simulink model "demo"  (Simulink 7.5)
settings: Solver=ode5  StartTime=0.0  StopTime=60  FixedStep=0.001  RelTol=1e-3
libraries: mathlib x58, logiclib x37, execlib x12, reglib x12, genlib x8, anallib x4
settings Model: Creator=jsobota  LastModifiedBy=jsobota
settings SimMechanicsCC: VisOnUpdateDiagram=on

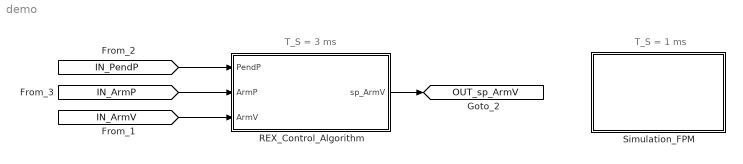
== system demo ==
  note: T_S = 3 ms
  note: T_S = 1 ms
  REX_Control_Algorithm : Subsystem  TreatAsAtomicUnit=on  SystemSampleTime=0.003
  Simulation_FPM : Subsystem  mask{g=9.81, r=0.3, l=0.23865, tau=0.06, rotate_sensor=-80*pi/180, alpha_pos0=0, alpha_vel0=0, beta_pos0=180*pi/180, beta_vel0=0}
      mask prompts: g "Gravity [m/s^2]"; r "Arm length [m]"; l "Pendulum length [m]"; tau "Velocity loop time constant"; rotate_sensor "Pendulum rotation sensor placement [rad]"; alpha_pos0 "Arm initial position [rad]"; alpha_vel0 "Arm initial velocity [rad/s]"; beta_pos0 "Pendulum initial position [rad]"; beta_vel0 "Pendulum initial velocity [rad/s]"
  tag scope: OUT_sp_ArmV=global
  wires:
  REX_Control_Algorithm/1(sp_ArmV) -> [OUT_sp_ArmV]
  [IN_PendP] -> REX_Control_Algorithm/1(PendP)
  [IN_ArmP] -> REX_Control_Algorithm/2(ArmP)
  [IN_ArmV] -> REX_Control_Algorithm/3(ArmV)

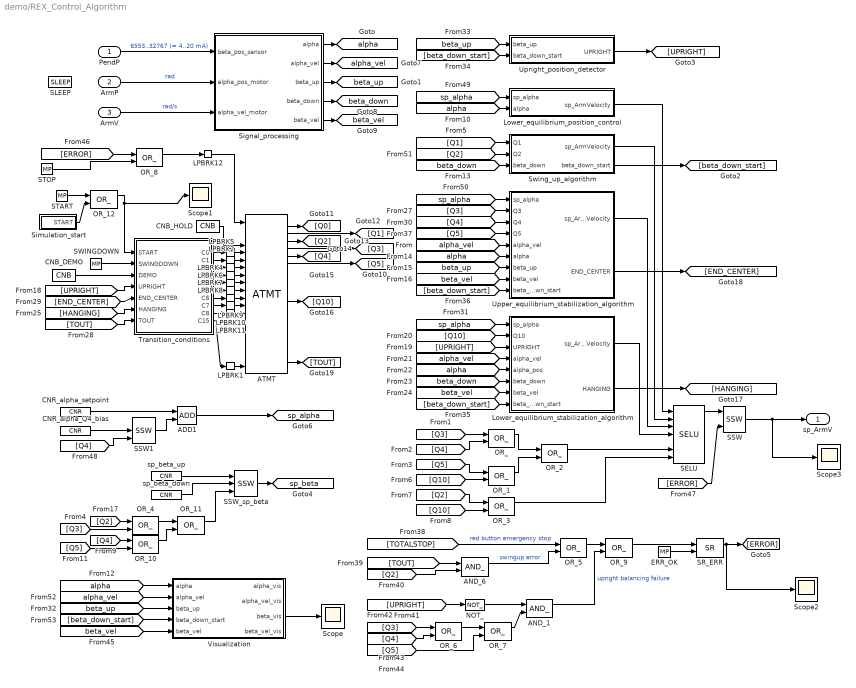
== system demo/REX_Control_Algorithm ==
  PendP : Inport
  ArmP : Inport  Port=2
  ArmV : Inport  Port=3
  ADD1 : mathlib/ADD  SystemSampleTime=-1
  AND_1 : logiclib/AND_  SystemSampleTime=-1
  AND_6 : logiclib/AND_  SystemSampleTime=-1
  ATMT : logiclib/ATMT  SystemSampleTime=-1  morestps=off  ntr=12  STT=[0 0 1;1 15 2;2 1 3;3 2 4;3 3 5;3 4 10;4 5 5;4 15 5;5 6 10;10 7 11;10 8 0;11 15 1]  touts=[0 0.5 1 20 10 10 0 0 0 0 5 5 0 0 0 0]
  CNB_DEMO : mathlib/CNB  SystemSampleTime=-1  YCN=on
  CNB_HOLD : mathlib/CNB  SystemSampleTime=-1  YCN=off
  CNR_alpha_Q4_bias : mathlib/CNR  SystemSampleTime=-1  ycn=3.1415
  CNR_alpha_setpoint : mathlib/CNR  SystemSampleTime=-1  ycn=0
  ERR_OK : genlib/MP  SystemSampleTime=-1  pwidth=0.01  BSTATE=off  RPTF=off
  LPBRK{1..2,4..12} (11 alike) : execlib/LPBRK
  Lower_equilibrium_position_control : Subsystem
      mask Type: REX sequence
  Lower_equilibrium_stabilization_algorithm : Subsystem
      mask Type: REX sequence
  NOT_ : logiclib/NOT_  SystemSampleTime=-1
  OR_{,1..12} (13 alike) : logiclib/OR_  SystemSampleTime=-1
  SELU : reglib/SELU  SystemSampleTime=-1  BINF=on
  SLEEP : execlib/SLEEP  SystemSampleTime=-1  ts=0
  SR_ERR : logiclib/SR  SystemSampleTime=-1
  SSW : reglib/SSW  SystemSampleTime=-1
  SSW1 : reglib/SSW  SystemSampleTime=-1
  SSW_sp_beta : reglib/SSW  SystemSampleTime=-1
  START : genlib/MP  SystemSampleTime=-1  pwidth=0.01  BSTATE=off  RPTF=off
  STOP : genlib/MP  SystemSampleTime=-1  pwidth=0.01  BSTATE=off  RPTF=off
  SWINGDOWN : genlib/MP  SystemSampleTime=-1  pwidth=0.01  BSTATE=off  RPTF=off
  Scope{,1..3} (4 alike) : Scope
      Scope settings: TimeRange=10  YMin=-4
      Scope1 settings: TimeRange=10  YMin=-4
      Scope2 settings: TimeRange=10  YMin=-4  SaveName=ScopeData2
      Scope3 settings: TimeRange=10  YMin=-4  SaveName=ScopeData3
  Signal_processing : Subsystem
      mask Type: REX sequence
  Simulation_start : Subsystem
  Swing_up_algorithm : Subsystem
      mask Type: REX sequence
  Transition_conditions : Subsystem
  Upper_equilibrium_stabilization_algorithm : Subsystem
      mask Type: REX sequence
  Upright_position_detector : Subsystem
  Visualization : Subsystem
  sp_beta_down : mathlib/CNR  SystemSampleTime=-1  ycn=3.1415
  sp_beta_up : mathlib/CNR  SystemSampleTime=-1  ycn=0
  sp_ArmV : Outport
  tag scope: alpha=global, alpha_vel=global, beta_down=global, beta_up=global, beta_vel=global, sp_alpha=global, sp_beta=global
  wires:
  ATMT/1 -> [Q0]
  ATMT/2 -> [Q1]
  ATMT/3 -> [Q2]
  ATMT/4 -> [Q3]
  ATMT/5 -> [Q4]
  ATMT/11 -> [Q10]
  ATMT/19 -> [TOUT]
  [alpha_vel] -> Upper_equilibrium_stabilization_algorithm/5(alpha_vel)
  [Q3] -> OR_/1
  [alpha] -> Lower_equilibrium_position_control/2(alpha)
  [beta_down] -> Swing_up_algorithm/3(beta_down)
  [alpha] -> Upper_equilibrium_stabilization_algorithm/6(alpha)
  [beta_up] -> Upper_equilibrium_stabilization_algorithm/7(beta_up)
  [beta_vel] -> Upper_equilibrium_stabilization_algorithm/8(beta_vel)
  [UPRIGHT] -> Lower_equilibrium_stabilization_algorithm/3(UPRIGHT)
  [Q4] -> OR_/2
  [Q10] -> Lower_equilibrium_stabilization_algorithm/2(Q10)
  [alpha_vel] -> Lower_equilibrium_stabilization_algorithm/4(alpha_vel)
  [alpha] -> Lower_equilibrium_stabilization_algorithm/5(alpha_pos)
  [beta_down] -> Lower_equilibrium_stabilization_algorithm/6(beta_down)
  [beta_vel] -> Lower_equilibrium_stabilization_algorithm/7(beta_vel)
  [Q3] -> Upper_equilibrium_stabilization_algorithm/2(Q3)
  [Q5] -> OR_1/1
  [Q10] -> OR_1/2
  [Q2] -> OR_3/1
  [Q10] -> OR_3/2
  ArmV/1 -> Signal_processing/3(alpha_vel_motor)  "rad/s"
  PendP/1 -> Signal_processing/1(beta_pos_sensor)  "6553..32767 (= 4..20 mA)"
  CNB_HOLD/1 -> ATMT/4
  LPBRK1/1 -> ATMT/20
  Lower_equilibrium_position_control/1(sp_ArmVelocity) -> SELU/1
  Lower_equilibrium_stabilization_algorithm/1(sp_ArmVelocity) -> SELU/4
  Lower_equilibrium_stabilization_algorithm/2(HANGING) -> [HANGING]
  OR_/1 -> OR_2/1
  OR_1/1 -> OR_2/2
  OR_2/1 -> SELU/6
  OR_3/1 -> SELU/7
  Signal_processing/1(alpha) -> [alpha]
  Signal_processing/2(alpha_vel) -> [alpha_vel]
  Signal_processing/3(beta_up) -> [beta_up]
  Signal_processing/4(beta_down) -> [beta_down]
  Signal_processing/5(beta_vel) -> [beta_vel]
  Swing_up_algorithm/1(sp_ArmVelocity) -> SELU/2
  Swing_up_algorithm/2(beta_down_start) -> [beta_down_start]
  Upper_equilibrium_stabilization_algorithm/1(sp_ArmVelocity) -> SELU/3
  ArmP/1 -> Signal_processing/2(alpha_pos_motor)  "rad"
  Upper_equilibrium_stabilization_algorithm/2(END_CENTER) -> [END_CENTER]
  [Q4] -> Upper_equilibrium_stabilization_algorithm/3(Q4)
  Upright_position_detector/1(UPRIGHT) -> [UPRIGHT]
  [beta_up] -> Upright_position_detector/1(beta_up)
  [beta_down_start] -> Upright_position_detector/2(beta_down_start)
  [beta_down_start] -> Lower_equilibrium_stabilization_algorithm/8(beta_down_start)
  [beta_down_start] -> Upper_equilibrium_stabilization_algorithm/9(beta_down_start)
  [Q5] -> Upper_equilibrium_stabilization_algorithm/4(Q5)
  [TOUT] -> AND_6/1
  [Q2] -> AND_6/2
  [UPRIGHT] -> NOT_/1
  [Q3] -> OR_6/1
  [Q4] -> OR_6/2
  [Q5] -> OR_7/2
  OR_6/1 -> OR_7/1
  OR_7/1 -> AND_1/2
  NOT_/1 -> AND_1/1
  AND_1/1 -> OR_9/2  "upright balancing failure"
  [TOTALSTOP] -> OR_5/1  "red button emergency stop"
  AND_6/1 -> OR_5/2  "swingup error"
  ERR_OK/1 -> SR_ERR/2
  SR_ERR/1 -> [ERROR], Scope2/1
  [ERROR] -> OR_8/1
  STOP/1 -> OR_8/2
  OR_8/1 -> LPBRK12/1
  SELU/1 -> SSW/1
  SSW/1 -> sp_ArmV/1, Scope3/1
  [ERROR] -> SSW/3
  CNR_alpha_setpoint/1 -> ADD1/1
  SSW1/1 -> ADD1/2
  [Q4] -> SSW1/3
  CNR_alpha_Q4_bias/1 -> SSW1/2
  ADD1/1 -> [sp_alpha]
  [sp_alpha] -> Lower_equilibrium_position_control/1(sp_alpha)
  [sp_alpha] -> Upper_equilibrium_stabilization_algorithm/1(sp_alpha)
  [Q1] -> Swing_up_algorithm/1(Q1)
  [Q2] -> Swing_up_algorithm/2(Q2)
  ATMT/6 -> [Q5]
  OR_5/1 -> OR_9/1
  OR_9/1 -> SR_ERR/1
  Transition_conditions/10(C15) -> LPBRK1/1
  CNB_DEMO/1 -> Transition_conditions/3(DEMO)
  SWINGDOWN/1 -> Transition_conditions/2(SWINGDOWN)
  START/1 -> OR_12/1
  [UPRIGHT] -> Transition_conditions/4(UPRIGHT)
  [END_CENTER] -> Transition_conditions/5(END_CENTER)
  [HANGING] -> Transition_conditions/6(HANGING)
  [TOUT] -> Transition_conditions/7(TOUT)
  Transition_conditions/1(C0) -> LPBRK5/1
  LPBRK5/1 -> ATMT/5
  Transition_conditions/2(C1) -> LPBRK2/1
  Transition_conditions/3(C2) -> LPBRK4/1
  Transition_conditions/4(C3) -> LPBRK6/1
  Transition_conditions/5(C4) -> LPBRK7/1
  Transition_conditions/6(C5) -> LPBRK8/1
  Transition_conditions/7(C6) -> LPBRK9/1
  Transition_conditions/8(C7) -> LPBRK10/1
  Transition_conditions/9(C8) -> LPBRK11/1
  LPBRK12/1 -> ATMT/1
  [sp_alpha] -> Lower_equilibrium_stabilization_algorithm/1(sp_alpha)
  Simulation_start/1(START) -> OR_12/2
  LPBRK2/1 -> ATMT/6
  LPBRK4/1 -> ATMT/7
  LPBRK6/1 -> ATMT/8
  LPBRK7/1 -> ATMT/9
  LPBRK8/1 -> ATMT/10
  LPBRK9/1 -> ATMT/11
  LPBRK10/1 -> ATMT/12
  LPBRK11/1 -> ATMT/13
  [alpha] -> Visualization/1(alpha)
  [alpha_vel] -> Visualization/2(alpha_vel)
  [beta_up] -> Visualization/3(beta_up)
  [beta_down_start] -> Visualization/4(beta_down_start)
  [beta_vel] -> Visualization/5(beta_vel)
  Visualization/3(beta_vis) -> Scope/1
  sp_beta_up/1 -> SSW_sp_beta/1
  sp_beta_down/1 -> SSW_sp_beta/2
  [Q2] -> OR_4/1
  [Q3] -> OR_4/2
  [Q4] -> OR_10/1
  [Q5] -> OR_10/2
  OR_4/1 -> OR_11/1
  OR_10/1 -> OR_11/2
  OR_11/1 -> SSW_sp_beta/3
  SSW_sp_beta/1 -> [sp_beta]
  OR_12/1 -> Transition_conditions/1(START), Scope1/1

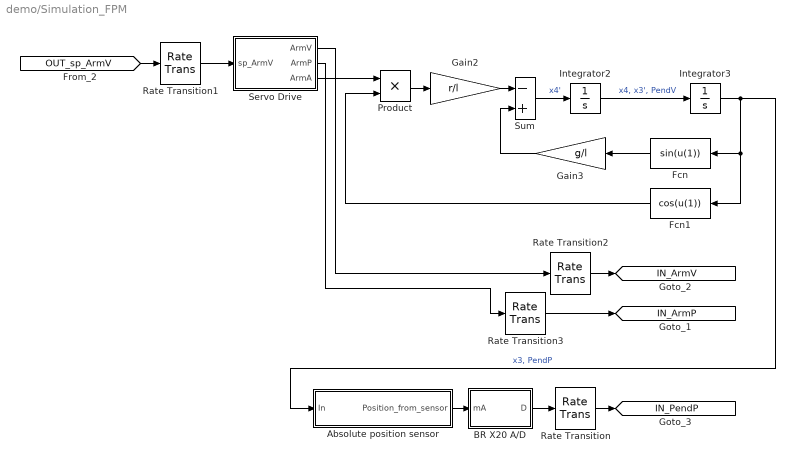
== system demo/Simulation_FPM ==
  Absolute position sensor : Subsystem
  BR X20 A/D : Subsystem
  Fcn : Fcn  Expr=sin(u(1))
  Fcn1 : Fcn  Expr=cos(u(1))
  Gain2 : Gain  Gain=r/l  ParameterDataType=fixdt(1, 16)  ParameterScaling=2^0  OutDataType=fixdt(1, 16)  OutScaling=2^0
  Gain3 : Gain  Gain=g/l  ParameterDataType=fixdt(1, 16)  ParameterScaling=2^0  OutDataType=fixdt(1, 16)  OutScaling=2^0
  Integrator2 : Integrator  InitialCondition=beta_vel0
  Integrator3 : Integrator  InitialCondition=beta_pos0
  Product : Product  OutDataType=fixdt(1, 16)  OutScaling=2^0  RndMeth=Zero
  Rate Transition : RateTransition  Integrity=off  OutPortSampleTimeOpt=Inherit  OutPortSampleTime=0.1
  Rate Transition1 : RateTransition  Integrity=off  Deterministic=off  OutPortSampleTimeOpt=Inherit
  Rate Transition2 : RateTransition  Integrity=off  OutPortSampleTimeOpt=Inherit  OutPortSampleTime=0.1
  Rate Transition3 : RateTransition  Integrity=off  OutPortSampleTimeOpt=Inherit  OutPortSampleTime=0.1
  Servo Drive : Subsystem
  Sum : Sum  Inputs=-+  OutDataType=fixdt(1, 16)  OutScaling=2^0
  tag scope: IN_ArmP=global, IN_ArmV=global, IN_PendP=global
  wires:
  Sum/1 -> Integrator2/1  "x4'"
  Integrator2/1 -> Integrator3/1  "x4, x3', PendV"
  Integrator3/1 -> Absolute position sensor/1(In), Fcn/1, Fcn1/1  "x3, PendP"
  Gain3/1 -> Sum/2
  Fcn/1 -> Gain3/1
  Fcn1/1 -> Product/2
  Product/1 -> Gain2/1
  Gain2/1 -> Sum/1
  Servo Drive/2(ArmP) -> Rate Transition3/1
  [OUT_sp_ArmV] -> Rate Transition1/1
  Rate Transition1/1 -> Servo Drive/1(sp_ArmV)
  Rate Transition/1 -> [IN_PendP]
  Rate Transition2/1 -> [IN_ArmV]
  Rate Transition3/1 -> [IN_ArmP]
  Servo Drive/1(ArmV) -> Rate Transition2/1
  Servo Drive/3(ArmA) -> Product/1
  Absolute position sensor/1(Position_from_sensor) -> BR X20 A/D/1(mA)
  BR X20 A/D/1(D) -> Rate Transition/1

== system demo/REX_Control_Algorithm/Lower_equilibrium_position_control ==
  sp_alpha : Inport
  alpha : Inport  Port=2
  GAIN_P_controller : mathlib/GAIN  SystemSampleTime=-1  k=2
  SUB : mathlib/SUB  SystemSampleTime=-1
  sp_ArmVelocity : Outport
  wires:
  GAIN_P_controller/1 -> sp_ArmVelocity/1
  SUB/1 -> GAIN_P_controller/1
  alpha/1 -> SUB/2
  sp_alpha/1 -> SUB/1

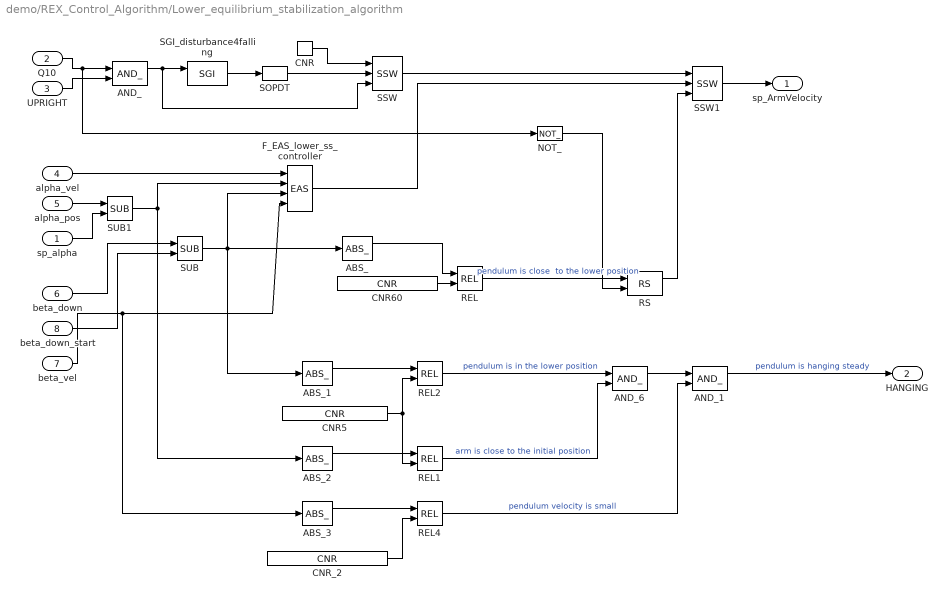
== system demo/REX_Control_Algorithm/Lower_equilibrium_stabilization_algorithm ==
  sp_alpha : Inport
  Q10 : Inport  Port=2
  UPRIGHT : Inport  Port=3
  alpha_vel : Inport  Port=4
  alpha_pos : Inport  Port=5
  beta_down : Inport  Port=6  OutDataType=sfix(16)  OutScaling=2^0
  beta_vel : Inport  Port=7  OutDataType=sfix(16)  OutScaling=2^0
  beta_down_start : Inport  Port=8  OutDataType=sfix(16)  OutScaling=2^0
  ABS_{,1..3} (4 alike) : mathlib/ABS_  SystemSampleTime=-1
  AND_ : logiclib/AND_  SystemSampleTime=-1
  AND_1 : logiclib/AND_  SystemSampleTime=-1
  AND_6 : logiclib/AND_  SystemSampleTime=-1
  CNR : mathlib/CNR  SystemSampleTime=-1  ycn=0
  CNR5 : mathlib/CNR  SystemSampleTime=-1  ycn=0.087266462599716
  CNR60 : mathlib/CNR  SystemSampleTime=-1  ycn=0.5
  CNR_2 : mathlib/CNR  SystemSampleTime=-1  ycn=0.0017453292519943
  F_EAS_lower_ss_controller : mathlib/EAS  SystemSampleTime=-1  a=6.12354219E-001  b=-4.25163230E-001  c=-2.53804417E+000  d=-3.30908089E-001  y0=0
  NOT_ : logiclib/NOT_  SystemSampleTime=-1
  REL{,1..2,4} (4 alike) : mathlib/REL  SystemSampleTime=-1  irel=3: less than (<)
  RS : logiclib/RS  SystemSampleTime=-1
  SGI_disturbance4falling : genlib/SGI  SystemSampleTime=-1  isig=4: RANDOM  amp=1  freq=1  phase=0  ifrunit=1: Hz  iphunit=1: degrees
  SOPDT : reglib/SOPDT  SystemSampleTime=-1  itf=2: Real poles  k0=1  tau=0  tau1=0.1  tau2=0.2  om=1  xi=1  pb0=1  pb1=1  pa0=1  pa1=1  del=0
  SSW : reglib/SSW  SystemSampleTime=-1
  SSW1 : reglib/SSW  SystemSampleTime=-1
  SUB : mathlib/SUB  SystemSampleTime=-1
  SUB1 : mathlib/SUB  SystemSampleTime=-1
  sp_ArmVelocity : Outport
  HANGING : Outport  Port=2
  wires:
  ABS_/1 -> REL/1
  ABS_1/1 -> REL2/1
  ABS_2/1 -> REL1/1
  ABS_3/1 -> REL4/1
  AND_/1 -> SGI_disturbance4falling/1, SSW/3
  AND_1/1 -> HANGING/1  "pendulum is hanging steady"
  AND_6/1 -> AND_1/1
  CNR/1 -> SSW/1
  CNR5/1 -> REL1/2, REL2/2
  CNR60/1 -> REL/2
  CNR_2/1 -> REL4/2
  F_EAS_lower_ss_controller/1 -> SSW1/2
  NOT_/1 -> RS/2
  Q10/1 -> AND_/1, NOT_/1
  REL/1 -> RS/1  "pendulum is close  to the lower position"
  REL1/1 -> AND_6/2  "arm is close to the initial position"
  REL2/1 -> AND_6/1  "pendulum is in the lower position"
  REL4/1 -> AND_1/2  "pendulum velocity is small"
  RS/1 -> SSW1/3
  SGI_disturbance4falling/1 -> SOPDT/1
  SOPDT/1 -> SSW/2
  SSW/1 -> SSW1/1
  SSW1/1 -> sp_ArmVelocity/1
  SUB/1 -> ABS_/1, ABS_1/1, F_EAS_lower_ss_controller/3
  UPRIGHT/1 -> AND_/2
  alpha_pos/1 -> SUB1/1
  alpha_vel/1 -> F_EAS_lower_ss_controller/1
  beta_down/1 -> SUB/1
  beta_down_start/1 -> SUB/2
  beta_vel/1 -> ABS_3/1, F_EAS_lower_ss_controller/4
  SUB1/1 -> ABS_2/1, F_EAS_lower_ss_controller/2
  sp_alpha/1 -> SUB1/2

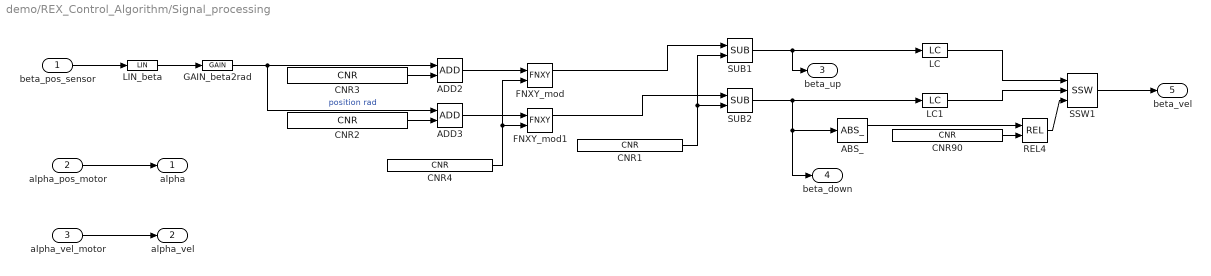
== system demo/REX_Control_Algorithm/Signal_processing ==
  beta_pos_sensor : Inport
  alpha_pos_motor : Inport  Port=2
  alpha_vel_motor : Inport  Port=3
  ABS_ : mathlib/ABS_  SystemSampleTime=-1
  ADD2 : mathlib/ADD  SystemSampleTime=-1
  ADD3 : mathlib/ADD  SystemSampleTime=-1
  CNR1 : mathlib/CNR  SystemSampleTime=-1  ycn=3.14159265358979
  CNR2 : mathlib/CNR  SystemSampleTime=-1  ycn=4.71238898038469
  CNR3 : mathlib/CNR  SystemSampleTime=-1  ycn=7.853981633974483
  CNR4 : mathlib/CNR  SystemSampleTime=-1  ycn=6.283185307179586
  CNR90 : mathlib/CNR  SystemSampleTime=-1  ycn=1.570796326794897
  FNXY_mod : mathlib/FNXY  SystemSampleTime=-1  ifn=2: fmod  yerr=0.0
  FNXY_mod1 : mathlib/FNXY  SystemSampleTime=-1  ifn=2: fmod  yerr=0.0
  GAIN_beta2rad : mathlib/GAIN  SystemSampleTime=-1  k=0.0175
  LC : reglib/LC  SystemSampleTime=-1  td=1  nd=30  ISSF=off
  LC1 : reglib/LC  SystemSampleTime=-1  td=1  nd=30  ISSF=off
  LIN_beta : mathlib/LIN  SystemSampleTime=-1  u1=6553  y1=5  u2=32767  y2=355
  REL4 : mathlib/REL  SystemSampleTime=-1  irel=3: less than (<)
  SSW1 : reglib/SSW  SystemSampleTime=-1
  SUB1 : mathlib/SUB  SystemSampleTime=-1
  SUB2 : mathlib/SUB  SystemSampleTime=-1
  alpha : Outport
  alpha_vel : Outport  Port=2
  beta_up : Outport  Port=3
  beta_down : Outport  Port=4
  beta_vel : Outport  Port=5
  wires:
  ABS_/1 -> REL4/1
  ADD2/1 -> FNXY_mod/1
  ADD3/1 -> FNXY_mod1/1
  CNR1/1 -> SUB1/2, SUB2/2
  CNR2/1 -> ADD3/2
  CNR3/1 -> ADD2/2
  CNR4/1 -> FNXY_mod/2, FNXY_mod1/2
  CNR90/1 -> REL4/2
  FNXY_mod/1 -> SUB1/1
  FNXY_mod1/1 -> SUB2/1
  GAIN_beta2rad/1 -> ADD2/1, ADD3/1  "position rad"
  LC/1 -> SSW1/1
  LC1/1 -> SSW1/2
  REL4/1 -> SSW1/3
  SSW1/1 -> beta_vel/1
  SUB1/1 -> LC/1, beta_up/1
  SUB2/1 -> ABS_/1, beta_down/1, LC1/1
  alpha_vel_motor/1 -> alpha_vel/1
  LIN_beta/1 -> GAIN_beta2rad/1
  beta_pos_sensor/1 -> LIN_beta/1
  alpha_pos_motor/1 -> alpha/1

== system demo/REX_Control_Algorithm/Simulation_start ==
  BIS : genlib/BIS  SystemSampleTime=-1  Y0=off  t1=5  t2=6  t3=0  t4=4  t5=5  t6=6  t7=7  t8=8  RPT=off
  START : Outport
  wires:
  BIS/1 -> START/1

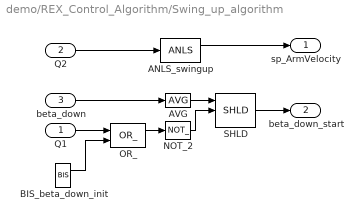
== system demo/REX_Control_Algorithm/Swing_up_algorithm ==
  Q1 : Inport
  Q2 : Inport  Port=2
  beta_down : Inport  Port=3  OutDataType=sfix(16)  OutScaling=2^0
  ANLS_swingup : genlib/ANLS  SystemSampleTime=-1  y0=-10  t1=0.226  y1=-10  t2=0.226  y2=10  t3=1  y3=10  t4=1  y4=0  RPT=off
  AVG : anallib/AVG  SystemSampleTime=-1  n=100
  BIS_beta_down_init : genlib/BIS  SystemSampleTime=-1  Y0=off  t1=1  t2=2  t3=0  t4=4  t5=5  t6=6  t7=7  t8=8  RPT=off
  NOT_2 : logiclib/NOT_  SystemSampleTime=-1
  OR_ : logiclib/OR_  SystemSampleTime=-1
  SHLD : anallib/SHLD  SystemSampleTime=-1  y0=0
  sp_ArmVelocity : Outport
  beta_down_start : Outport  Port=2
  wires:
  ANLS_swingup/1 -> sp_ArmVelocity/1
  AVG/1 -> SHLD/1
  NOT_2/1 -> SHLD/2
  Q2/1 -> ANLS_swingup/1
  SHLD/1 -> beta_down_start/1
  beta_down/1 -> AVG/1
  Q1/1 -> OR_/1
  BIS_beta_down_init/1 -> OR_/2
  OR_/1 -> NOT_2/1

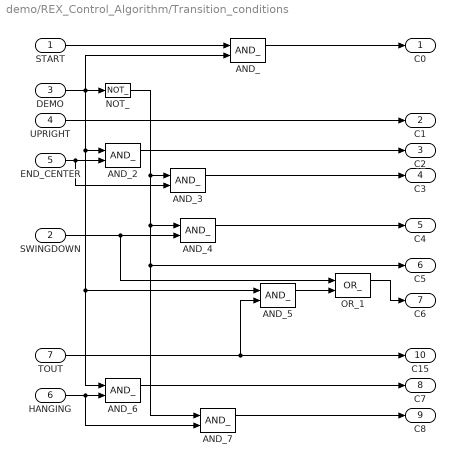
== system demo/REX_Control_Algorithm/Transition_conditions ==
  START : Inport
  SWINGDOWN : Inport  Port=2
  DEMO : Inport  Port=3
  UPRIGHT : Inport  Port=4
  END_CENTER : Inport  Port=5
  HANGING : Inport  Port=6
  TOUT : Inport  Port=7
  AND_{,2..7} (7 alike) : logiclib/AND_  SystemSampleTime=-1
  NOT_ : logiclib/NOT_  SystemSampleTime=-1
  OR_1 : logiclib/OR_  SystemSampleTime=-1
  C0 : Outport
  C1 : Outport  Port=2
  C2 : Outport  Port=3
  C3 : Outport  Port=4
  C4 : Outport  Port=5
  C5 : Outport  Port=6
  C6 : Outport  Port=7
  C7 : Outport  Port=8
  C8 : Outport  Port=9
  C15 : Outport  Port=10
  wires:
  START/1 -> AND_/1
  DEMO/1 -> AND_/2, NOT_/1, AND_2/1, AND_5/1, AND_6/1
  AND_/1 -> C0/1
  NOT_/1 -> AND_3/1, AND_4/1, C5/1, AND_7/1
  TOUT/1 -> C15/1, AND_5/2
  UPRIGHT/1 -> C1/1
  END_CENTER/1 -> AND_2/2, AND_3/2
  AND_2/1 -> C2/1
  AND_3/1 -> C3/1
  SWINGDOWN/1 -> AND_4/2, OR_1/1
  AND_4/1 -> C4/1
  AND_5/1 -> OR_1/2
  OR_1/1 -> C6/1
  HANGING/1 -> AND_6/2, AND_7/2
  AND_6/1 -> C7/1
  AND_7/1 -> C8/1

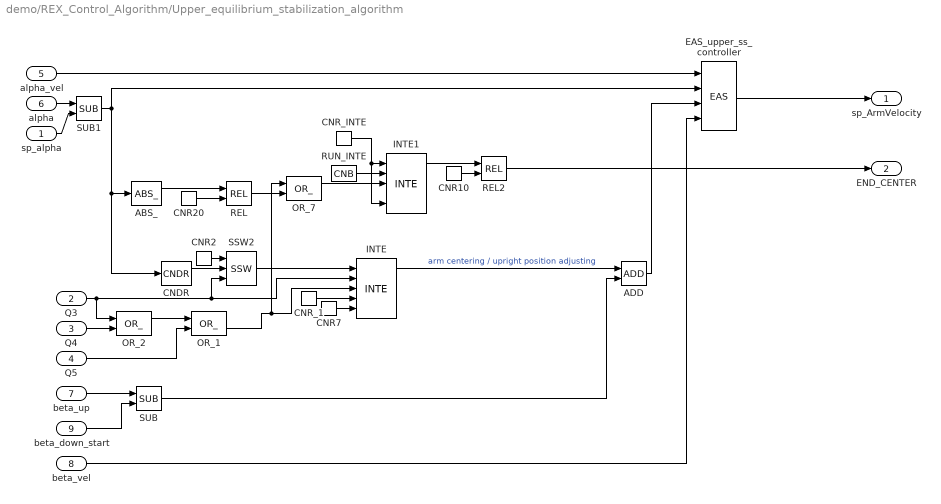
== system demo/REX_Control_Algorithm/Upper_equilibrium_stabilization_algorithm ==
  sp_alpha : Inport
  Q3 : Inport  Port=2
  Q4 : Inport  Port=3
  Q5 : Inport  Port=4
  alpha_vel : Inport  Port=5
  alpha : Inport  Port=6
  beta_up : Inport  Port=7  OutDataType=sfix(16)  OutScaling=2^0
  beta_vel : Inport  Port=8  OutDataType=sfix(16)  OutScaling=2^0
  beta_down_start : Inport  Port=9  OutDataType=sfix(16)  OutScaling=2^0
  ABS_ : mathlib/ABS_  SystemSampleTime=-1
  ADD : mathlib/ADD  SystemSampleTime=-1
  CNDR : reglib/CNDR  SystemSampleTime=-1  n=6  SATF=on  up=[-1.5708 -0.7854 -0.0523 0.0523 0.7854 1.5708]  yp=[-0.12 -0.04 0 0 0.04 0.12]
  CNR10 : mathlib/CNR  SystemSampleTime=-1  ycn=20
  CNR2 : mathlib/CNR  SystemSampleTime=-1  ycn=0
  CNR20 : mathlib/CNR  SystemSampleTime=-1  ycn=0.349065850398866
  CNR7 : mathlib/CNR  SystemSampleTime=-1  ycn=20
  CNR_1 : mathlib/CNR  SystemSampleTime=-1  ycn=0
  CNR_INTE : mathlib/CNR  SystemSampleTime=-1  ycn=1
  EAS_upper_ss_controller : mathlib/EAS  SystemSampleTime=-1  a=1.173059924  b=.1334856247  c=4.815526508  d=.7295211418  y0=0
  INTE : anallib/INTE  SystemSampleTime=-1  ymin=-1  ymax=1
  INTE1 : anallib/INTE  SystemSampleTime=-1  ymin=0  ymax=30
  OR_1 : logiclib/OR_  SystemSampleTime=-1
  OR_2 : logiclib/OR_  SystemSampleTime=-1
  OR_7 : logiclib/OR_  SystemSampleTime=-1
  REL : mathlib/REL  SystemSampleTime=-1  irel=4: greater than (>)
  REL2 : mathlib/REL  SystemSampleTime=-1  irel=4: greater than (>)
  RUN_INTE : mathlib/CNB  SystemSampleTime=-1  YCN=on
  SSW2 : reglib/SSW  SystemSampleTime=-1
  SUB : mathlib/SUB  SystemSampleTime=-1
  SUB1 : mathlib/SUB  SystemSampleTime=-1
  sp_ArmVelocity : Outport
  END_CENTER : Outport  Port=2
  wires:
  ABS_/1 -> REL/1
  ADD/1 -> EAS_upper_ss_controller/3
  CNDR/1 -> SSW2/2
  CNR10/1 -> REL2/2
  CNR2/1 -> SSW2/1
  CNR20/1 -> REL/2
  CNR7/1 -> INTE/5
  CNR_1/1 -> INTE/4
  CNR_INTE/1 -> INTE1/1, INTE1/5
  EAS_upper_ss_controller/1 -> sp_ArmVelocity/1
  INTE/1 -> ADD/1  "arm centering / upright position adjusting"
  INTE1/1 -> REL2/1
  OR_1/2 -> INTE/3, OR_7/1
  OR_7/1 -> INTE1/3
  Q3/1 -> SSW2/3, INTE/2, OR_2/1
  REL/1 -> OR_7/2
  RUN_INTE/1 -> INTE1/2
  SSW2/1 -> INTE/1
  SUB/1 -> ADD/2
  SUB1/1 -> ABS_/1, CNDR/1, EAS_upper_ss_controller/2
  alpha_vel/1 -> EAS_upper_ss_controller/1
  beta_down_start/1 -> SUB/2
  beta_up/1 -> SUB/1
  beta_vel/1 -> EAS_upper_ss_controller/4
  REL2/1 -> END_CENTER/1
  Q4/1 -> OR_2/2
  Q5/1 -> OR_1/2
  OR_2/1 -> OR_1/1
  alpha/1 -> SUB1/1
  sp_alpha/1 -> SUB1/2

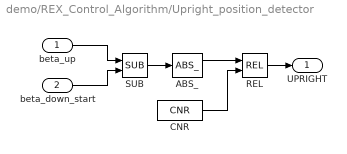
== system demo/REX_Control_Algorithm/Upright_position_detector ==
  beta_up : Inport
  beta_down_start : Inport  Port=2
  ABS_ : mathlib/ABS_  SystemSampleTime=-1
  CNR : mathlib/CNR  SystemSampleTime=-1  ycn=0.9
  REL : mathlib/REL  SystemSampleTime=-1  irel=3: less than (<)
  SUB : mathlib/SUB  SystemSampleTime=-1
  UPRIGHT : Outport
  wires:
  ABS_/1 -> REL/1
  CNR/1 -> REL/2
  SUB/1 -> ABS_/1
  beta_up/1 -> SUB/1
  REL/1 -> UPRIGHT/1
  beta_down_start/1 -> SUB/2

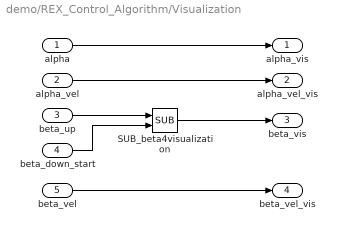
== system demo/REX_Control_Algorithm/Visualization ==
  alpha : Inport
  alpha_vel : Inport  Port=2
  beta_up : Inport  Port=3
  beta_down_start : Inport  Port=4
  beta_vel : Inport  Port=5
  SUB_beta4visualization : mathlib/SUB  SystemSampleTime=-1
  alpha_vis : Outport
  alpha_vel_vis : Outport  Port=2
  beta_vis : Outport  Port=3
  beta_vel_vis : Outport  Port=4
  wires:
  beta_up/1 -> SUB_beta4visualization/1
  beta_down_start/1 -> SUB_beta4visualization/2
  alpha/1 -> alpha_vis/1
  SUB_beta4visualization/1 -> beta_vis/1
  beta_vel/1 -> beta_vel_vis/1
  alpha_vel/1 -> alpha_vel_vis/1

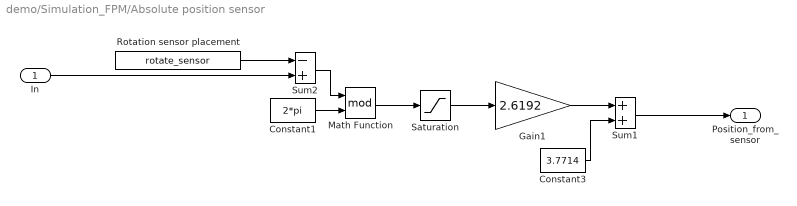
== system demo/Simulation_FPM/Absolute position sensor ==
  In : Inport
  Constant1 : Constant  Value=2*pi  OutDataType=fixdt(1, 16)  OutScaling=2^0
  Constant3 : Constant  Value=3.7714  OutDataType=fixdt(1, 16)  OutScaling=2^0
  Gain1 : Gain  Gain=2.6192  ParameterDataType=fixdt(1, 16)  ParameterScaling=2^0  OutDataType=fixdt(1, 16)  OutScaling=2^0
  Math Function : Math  Operator=mod  OutDataType=fixdt(1, 16)  OutScaling=2^0  SaturateOnIntegerOverflow=on
  Rotation sensor placement : Constant  Value=rotate_sensor  OutDataType=fixdt(1, 16)  OutScaling=2^0
  Saturation : Saturate  UpperLimit=355*pi/180  LowerLimit=5*pi/180  OutDataType=fixdt(1, 16)  OutScaling=2^0
  Sum1 : Sum  OutDataType=fixdt(1, 16)  OutScaling=2^0
  Sum2 : Sum  Inputs=-+  OutDataType=fixdt(1, 16)  OutScaling=2^0
  Position_from_sensor : Outport
  wires:
  Sum2/1 -> Math Function/1
  Rotation sensor placement/1 -> Sum2/1
  Math Function/1 -> Saturation/1
  Saturation/1 -> Gain1/1
  Constant1/1 -> Math Function/2
  In/1 -> Sum2/2
  Gain1/1 -> Sum1/1
  Constant3/1 -> Sum1/2
  Sum1/1 -> Position_from_sensor/1

== system demo/Simulation_FPM/BR X20 A/D ==
  mA : Inport
  Gain : Gain  Gain=1638.25  ParameterDataType=fixdt(1, 16)  ParameterScaling=2^0  OutDataType=fixdt(1, 16)  OutScaling=2^0
  D : Outport
  wires:
  mA/1 -> Gain/1
  Gain/1 -> D/1

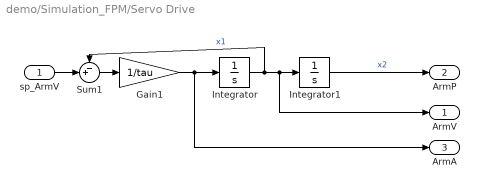
== system demo/Simulation_FPM/Servo Drive ==
  sp_ArmV : Inport
  Gain1 : Gain  Gain=1/tau  ParameterDataType=fixdt(1, 16)  ParameterScaling=2^0  OutDataType=fixdt(1, 16)  OutScaling=2^0
  Integrator : Integrator  InitialCondition=alpha_vel0
  Integrator1 : Integrator  InitialCondition=alpha_pos0
  Sum1 : Sum  Inputs=-+|  OutDataType=fixdt(1, 16)  OutScaling=2^0
  ArmV : Outport
  ArmP : Outport  Port=2
  ArmA : Outport  Port=3
  wires:
  Sum1/1 -> Gain1/1
  Integrator/1 -> Sum1/1, ArmV/1, Integrator1/1  "x1"
  Gain1/1 -> Integrator/1, ArmA/1
  Integrator1/1 -> ArmP/1  "x2"
  sp_ArmV/1 -> Sum1/2
